simulink model "AutomatedManualTransmission"  (R2026b)
settings: Solver=VariableStepAuto
undefined symbols (not defined in the file): PlntDriveshftDamp, PlntDriveshftStiff, PlntTransCltchRadius, PlntTransEffTempBpt, PlntTransGearRatioVect
libraries: autolibtransamt x1, autolibsharedcoupling x1
settings Model: ModifiedByFormat=The MathWorks, Inc.  Creator=The MathWorks, Inc.  LastModifiedBy=The MathWorks, Inc.

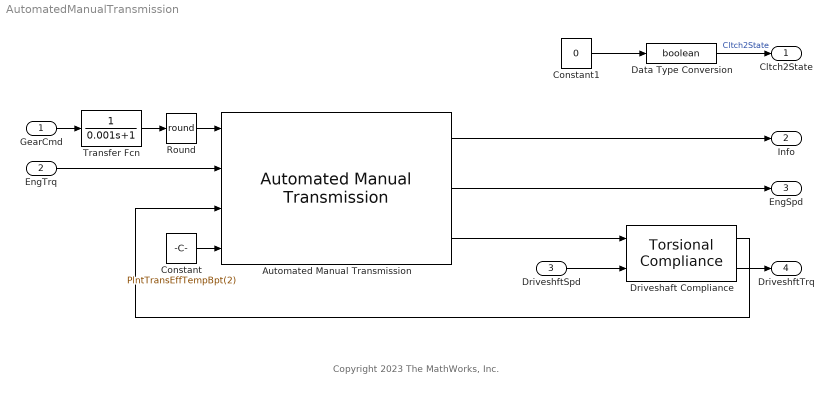
== system AutomatedManualTransmission ==
  note: Copyright 2023 The MathWorks, Inc.
  GearCmd : Inport
  EngTrq : Inport  Port=2
  DriveshftSpd : Inport  Port=3
  Automated Manual Transmission : autolibtransamt/Automated Manual Transmission  VariantControl=1  cntrlType=Ideal integrated controller  TransEffModelPopup=Gear, input torque, input speed, and temperature  Jin=PlntTransInInertia  bin=PlntTransInDamp  omegain_o=PlntTransInitInVel  G=PlntTransGearNumVect  Trq_bpts=PlntTransEffTrqBpt  omega_bpts=PlntTransEffSpdBpt  Temp_bpts=PlntTransEffTempBpt  N=PlntTransGearRatioVect  Jout=PlntTransInertiaVect  bout=PlntTransDampVect  eta=PlntTransEffVect  eta_tbl=PlntTransEffTbl  omegaout_o=PlntTransInitOutVel  G_o=PlntTransInitGear  tauc=PlntTransCltchPrsTimeCnst  ts=PlntTransCltchSyncTime  tc=PlntTransCltchTime  R=PlntTransCltchRadius  K_c=PlntTransCltchForceGain  mus=PlntTransCltchStatFric  muk=PlntTransCltchKinFric  ClutchLocked=off  SynchLocked=off  maxAbsSpd=5e3
  Constant : Constant  Value=PlntTransEffTempBpt(2)  SampleTime=-1
  Constant1 : Constant  Value=0  SampleTime=-1
  Data Type Conversion : DataTypeConversion  OutDataTypeStr=boolean  SaturateOnIntegerOverflow=off  RndMeth=Floor
  Driveshaft Compliance : autolibsharedcoupling/Torsional Compliance  port_config=Simulink  extInfo=off  k=PlntDriveshftStiff  b=PlntDriveshftDamp  theta_o=PlntDriveshftInitDeflect  domega_o=PlntDriveshftInitVel  omega_c=PlntDriveshftDampCutoffFreq  blkID=0  aMode=1
  Round : Rounding  Operator=round
  Transfer Fcn : TransferFcn  Denominator=[0.001 1]
  Cltch2State : Outport  VectorParamsAs1DForOutWhenUnconnected=off
  Info : Outport  Port=2  VectorParamsAs1DForOutWhenUnconnected=off
  EngSpd : Outport  Port=3  VectorParamsAs1DForOutWhenUnconnected=off
  DriveshftTrq : Outport  Port=4  VectorParamsAs1DForOutWhenUnconnected=off
  wires:
  DriveshftSpd/1 -> Driveshaft Compliance/2
  EngTrq/1 -> Automated Manual Transmission/2
  Automated Manual Transmission/1 -> Info/1
  Driveshaft Compliance/1 -> Automated Manual Transmission/3
  Automated Manual Transmission/3 -> Driveshaft Compliance/1
  Constant1/1 -> Data Type Conversion/1
  Driveshaft Compliance/2 -> DriveshftTrq/1
  Automated Manual Transmission/2 -> EngSpd/1
  GearCmd/1 -> Transfer Fcn/1
  Constant/1 -> Automated Manual Transmission/4
  Round/1 -> Automated Manual Transmission/1
  Transfer Fcn/1 -> Round/1
  Data Type Conversion/1 -> Cltch2State/1  "Cltch2State"
